simulink model "Channelizer_HLS_testbench"  (R2024a)
settings: Solver=VariableStepAuto  StartTime=0.0  StopTime=512  RelTol=1e-3
undefined symbols (not defined in the file): cyclicshift, permutei, permuteo, S, vsva2197, xcvc1902
libraries: aieUtilities x71, dspsrcs4 x23, hlsBasic x3, vmcUtilities x1
settings Model: Creator=robg  LastModifiedBy=robg
settings DebuggingCC: UnconnectedInputMsg=warning  UnconnectedOutputMsg=warning  UnconnectedLineMsg=warning
settings ModelReferenceCC: EnableRefExpFcnMdlSchedulingChecks=on
settings RTWCC: GPUComputeCapability=3.5  DLArmComputeVersion=19.05

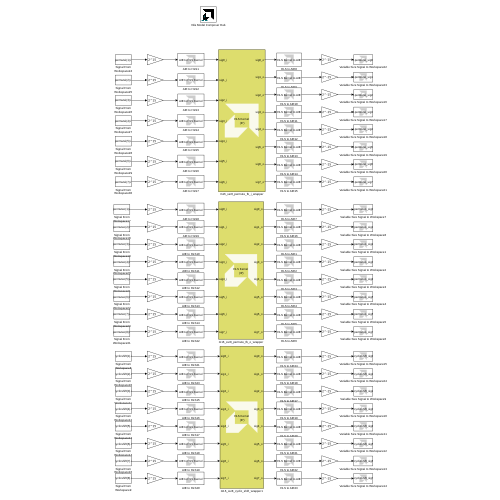
[thumbnail: Simulink's stored preview of the top-level diagram]
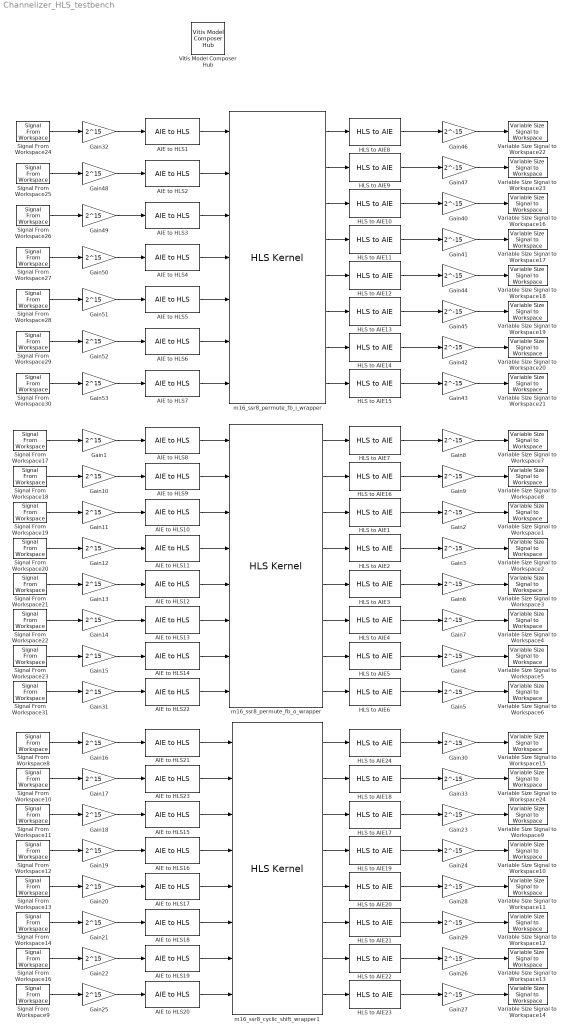
== system Channelizer_HLS_testbench ==
  AIE to HLS{1..23} (23 alike) : aieUtilities/AIE to HLS  OutputType=ufix128  OutputSize=1  AllowMultiRate=off  InputType=int8
  Gain{1,10..22,25,31..32,48..53} (23 alike) : Gain  Gain=2^15  OutDataTypeStr=int16
  Gain{2..9,23..24,26..30,33,40..47} (24 alike) : Gain  Gain=2^-15  OutDataTypeStr=double
  HLS to AIE{1..24} (24 alike) : aieUtilities/HLS to AIE  OutputType=cint16  OutputSize=4  AllowMultiRate=off  InputType=cint16
  Signal From Workspace10 : dspsrcs4/Signal From Workspace  X=cyclicshift(2).i  Ts=1  nsamps=4  OutputAfterFinalValue=Setting to zero  ignoreOrWarnInputAndFrameLengths=off  OutputFrames=off
  Signal From Workspace11 : dspsrcs4/Signal From Workspace  X=cyclicshift(3).i  Ts=1  nsamps=4  OutputAfterFinalValue=Setting to zero  ignoreOrWarnInputAndFrameLengths=off  OutputFrames=off
  Signal From Workspace12 : dspsrcs4/Signal From Workspace  X=cyclicshift(4).i  Ts=1  nsamps=4  OutputAfterFinalValue=Setting to zero  ignoreOrWarnInputAndFrameLengths=off  OutputFrames=off
  Signal From Workspace13 : dspsrcs4/Signal From Workspace  X=cyclicshift(5).i  Ts=1  nsamps=4  OutputAfterFinalValue=Setting to zero  ignoreOrWarnInputAndFrameLengths=off  OutputFrames=off
  Signal From Workspace14 : dspsrcs4/Signal From Workspace  X=cyclicshift(6).i  Ts=1  nsamps=4  OutputAfterFinalValue=Setting to zero  ignoreOrWarnInputAndFrameLengths=off  OutputFrames=off
  Signal From Workspace16 : dspsrcs4/Signal From Workspace  X=cyclicshift(7).i  Ts=1  nsamps=4  OutputAfterFinalValue=Setting to zero  ignoreOrWarnInputAndFrameLengths=off  OutputFrames=off
  Signal From Workspace17 : dspsrcs4/Signal From Workspace  X=permuteo(1).i  Ts=1  nsamps=4  OutputAfterFinalValue=Setting to zero  ignoreOrWarnInputAndFrameLengths=off  OutputFrames=off
  Signal From Workspace18 : dspsrcs4/Signal From Workspace  X=permuteo(2).i  Ts=1  nsamps=4  OutputAfterFinalValue=Setting to zero  ignoreOrWarnInputAndFrameLengths=off  OutputFrames=off
  Signal From Workspace19 : dspsrcs4/Signal From Workspace  X=permuteo(3).i  Ts=1  nsamps=4  OutputAfterFinalValue=Setting to zero  ignoreOrWarnInputAndFrameLengths=off  OutputFrames=off
  Signal From Workspace20 : dspsrcs4/Signal From Workspace  X=permuteo(4).i  Ts=1  nsamps=4  OutputAfterFinalValue=Setting to zero  ignoreOrWarnInputAndFrameLengths=off  OutputFrames=off
  Signal From Workspace21 : dspsrcs4/Signal From Workspace  X=permuteo(5).i  Ts=1  nsamps=4  OutputAfterFinalValue=Setting to zero  ignoreOrWarnInputAndFrameLengths=off  OutputFrames=off
  Signal From Workspace22 : dspsrcs4/Signal From Workspace  X=permuteo(6).i  Ts=1  nsamps=4  OutputAfterFinalValue=Setting to zero  ignoreOrWarnInputAndFrameLengths=off  OutputFrames=off
  Signal From Workspace23 : dspsrcs4/Signal From Workspace  X=permuteo(7).i  Ts=1  nsamps=4  OutputAfterFinalValue=Setting to zero  ignoreOrWarnInputAndFrameLengths=off  OutputFrames=off
  Signal From Workspace24 : dspsrcs4/Signal From Workspace  X=permutei(1).i  Ts=1  nsamps=4  OutputAfterFinalValue=Setting to zero  ignoreOrWarnInputAndFrameLengths=off  OutputFrames=off
  Signal From Workspace25 : dspsrcs4/Signal From Workspace  X=permutei(2).i  Ts=1  nsamps=4  OutputAfterFinalValue=Setting to zero  ignoreOrWarnInputAndFrameLengths=off  OutputFrames=off
  Signal From Workspace26 : dspsrcs4/Signal From Workspace  X=permutei(3).i  Ts=1  nsamps=4  OutputAfterFinalValue=Setting to zero  ignoreOrWarnInputAndFrameLengths=off  OutputFrames=off
  Signal From Workspace27 : dspsrcs4/Signal From Workspace  X=permutei(4).i  Ts=1  nsamps=4  OutputAfterFinalValue=Setting to zero  ignoreOrWarnInputAndFrameLengths=off  OutputFrames=off
  Signal From Workspace28 : dspsrcs4/Signal From Workspace  X=permutei(5).i  Ts=1  nsamps=4  OutputAfterFinalValue=Setting to zero  ignoreOrWarnInputAndFrameLengths=off  OutputFrames=off
  Signal From Workspace29 : dspsrcs4/Signal From Workspace  X=permutei(6).i  Ts=1  nsamps=4  OutputAfterFinalValue=Setting to zero  ignoreOrWarnInputAndFrameLengths=off  OutputFrames=off
  Signal From Workspace30 : dspsrcs4/Signal From Workspace  X=permutei(7).i  Ts=1  nsamps=4  OutputAfterFinalValue=Setting to zero  ignoreOrWarnInputAndFrameLengths=off  OutputFrames=off
  Signal From Workspace31 : dspsrcs4/Signal From Workspace  X=permuteo(8).i  Ts=1  nsamps=4  OutputAfterFinalValue=Setting to zero  ignoreOrWarnInputAndFrameLengths=off  OutputFrames=off
  Signal From Workspace8 : dspsrcs4/Signal From Workspace  X=cyclicshift(1).i  Ts=1  nsamps=4  OutputAfterFinalValue=Setting to zero  ignoreOrWarnInputAndFrameLengths=off  OutputFrames=off
  Signal From Workspace9 : dspsrcs4/Signal From Workspace  X=cyclicshift(8).i  Ts=1  nsamps=4  OutputAfterFinalValue=Setting to zero  ignoreOrWarnInputAndFrameLengths=off  OutputFrames=off
  Variable Size Signal to Workspace1 : aieUtilities/Variable Size Signal to Workspace  VariableNameMask=permuteo_sig2_o
  Variable Size Signal to Workspace10 : aieUtilities/Variable Size Signal to Workspace  VariableNameMask=cyclicshift_sig3_o
  Variable Size Signal to Workspace11 : aieUtilities/Variable Size Signal to Workspace  VariableNameMask=cyclicshift_sig4_o
  Variable Size Signal to Workspace12 : aieUtilities/Variable Size Signal to Workspace  VariableNameMask=cyclicshift_sig5_o
  Variable Size Signal to Workspace13 : aieUtilities/Variable Size Signal to Workspace  VariableNameMask=cyclicshift_sig6_o
  Variable Size Signal to Workspace14 : aieUtilities/Variable Size Signal to Workspace  VariableNameMask=cyclicshift_sig7_o
  Variable Size Signal to Workspace15 : aieUtilities/Variable Size Signal to Workspace  VariableNameMask=cyclicshift_sig0_o
  Variable Size Signal to Workspace16 : aieUtilities/Variable Size Signal to Workspace  VariableNameMask=permutei_sig2_o
  Variable Size Signal to Workspace17 : aieUtilities/Variable Size Signal to Workspace  VariableNameMask=permutei_sig3_o
  Variable Size Signal to Workspace18 : aieUtilities/Variable Size Signal to Workspace  VariableNameMask=permutei_sig4_o
  Variable Size Signal to Workspace19 : aieUtilities/Variable Size Signal to Workspace  VariableNameMask=permutei_sig5_o
  Variable Size Signal to Workspace2 : aieUtilities/Variable Size Signal to Workspace  VariableNameMask=permuteo_sig3_o
  Variable Size Signal to Workspace20 : aieUtilities/Variable Size Signal to Workspace  VariableNameMask=permutei_sig6_o
  Variable Size Signal to Workspace21 : aieUtilities/Variable Size Signal to Workspace  VariableNameMask=permutei_sig7_o
  Variable Size Signal to Workspace22 : aieUtilities/Variable Size Signal to Workspace  VariableNameMask=permutei_sig0_o
  Variable Size Signal to Workspace23 : aieUtilities/Variable Size Signal to Workspace  VariableNameMask=permutei_sig1_o
  Variable Size Signal to Workspace24 : aieUtilities/Variable Size Signal to Workspace  VariableNameMask=cyclicshift_sig1_o
  Variable Size Signal to Workspace3 : aieUtilities/Variable Size Signal to Workspace  VariableNameMask=permuteo_sig4_o
  Variable Size Signal to Workspace4 : aieUtilities/Variable Size Signal to Workspace  VariableNameMask=permuteo_sig5_o
  Variable Size Signal to Workspace5 : aieUtilities/Variable Size Signal to Workspace  VariableNameMask=permuteo_sig6_o
  Variable Size Signal to Workspace6 : aieUtilities/Variable Size Signal to Workspace  VariableNameMask=permuteo_sig7_o
  Variable Size Signal to Workspace7 : aieUtilities/Variable Size Signal to Workspace  VariableNameMask=permuteo_sig0_o
  Variable Size Signal to Workspace8 : aieUtilities/Variable Size Signal to Workspace  VariableNameMask=permuteo_sig1_o
  Variable Size Signal to Workspace9 : aieUtilities/Variable Size Signal to Workspace  VariableNameMask=cyclicshift_sig2_o
  Vitis Model Composer Hub : vmcUtilities/Vitis Model Composer Hub  Tag=genX  CodeGeneration=off  StartColumn=1  NumberOfColumns=1  TargetDirectory=./code  exportDesign=off  analyzeDesign=off  validateDesignOnHw=off  ExportType=AI Engines  IpVendor=xilinx.com  IpLibrary=hls  IpVersion=1.0  IpHWLanguage=Verilog  AieCompilerOptions={}  AieSimulatorOptions={}  CreateTestbench=off  TestbenchStackSize=10  RunRtlSim=off  RunCSim=off  RunAieSim=off  AieSimTimeout=50000  RunAieSimProfiling=off  LaunchVitisAnalyzer=off  PlotOutput=off  RunX86Sim=off  X86SimTimeout=10  GenHwImage=off  GenLibadfXo=off  GenHwValidationCode=off  PlatformType=Not Specified  HwSystemType=Baremetal  HwValidationTarget=hw  ProjDevice=xcvc1902-vsva2197-1LP-e-S  ProjDevicePart=xcvc1902-vsva2197-1LP-e-S  AIEType=AIE  SamplePeriod=-1  ClockFrequency=200  DataPathParallelism=1  xilinxfamily=versalaicore  part=xcvc1902  speed=-1LP-e-S  package=vsva2197  directory=./netlist  testbench=off  incr_netlist=off  synthesis_tool=Vivado  clock_wrapper=Clock Enables  dbl_ovrd=According to Block Masks  dcm_input_clock_period=10  sysclk_period=10  simulink_period=1  eval_field=0  LogFileName=''  NThreads=4
  m16_ssr8_cyclic_shift_wrapper1 : hlsBasic/HLS Kernel  PortNames={'return'; 'sig0_i'; 'sig1_i'; 'sig2_i'; 'sig3_i'; 'sig4_i'; 'sig5_i'; 'sig6_i'; 'sig7_i'; 'sig0_o'; 'sig1_o'; 'sig2_o'; 'sig3_o'; 'sig4_o'; 'sig5_o'; 'sig6_o'; 'sig7_o'}  PortSerializedTypes={'{Bv}'; '{R{Thls::stream{2{t{Tap_uint{1{t{}128}}}}{t{}0}}}}'; '{R{Thls::stream{2{t{Tap_uint{1{t{}128}}}}{t{}0}}}}'; '{R{Thls::stream{2{t{Tap_uint{1{t{}128}}}}{t{}0}}}}'; '{R{Thls::stream{2{t{Tap_uint{1{t{}128}}}}{t{}0}}}}'; '{R{Thls::stream{2{t{Tap_uint{1{t{}128}}}}{t{}0}}}}'; '{R{Thls::stream{2{t{Tap_uint{1{t{}128}}}}{t{}0}}}}'; '{R{Thls::stream{2{t{Tap_uint{1{t{}128}}}}{t{}0}}}}'; '{R{Thls::stream{2{t{Tap_uint{1{t{}128}}}}{t{}0}}}}'; '{R{Thls::stream{2{t{Tap_uint{1{t{}128}}}}{t{}0}}}}'; '{R{Thls::stream{2{t{Tap_uint{1{t{}128}}}}{t{}0}}}}'; '{R{Thls::stream{2{t{Tap_uint{1{t{}128}}}}{t{}0}}}}'; '{R{Thls::stream{2{t{Tap_uint{1{t{}128}}}}{t{}0}}}}'; '{R{Thls::stream{2{t{Tap_uint{1{t{}128}}}}{t{}0}}}}'; '{R{Thls::stream{2{t{Tap_uint{1{t{}128}}}}{t{}0}}}}'; '{R{Thls::stream{2{t{Tap_uint{1{t{}128}}}}{t{}0}}}}'; '{R{Thls::stream{2{t{Tap_uint{1{t{}128}}}}{t{}0}}}}'}  FunctionTemplateSpecKind=none  FunctionTemplateParamNames={}  FunctionTemplateParamKinds={}  FunctionTemplateParamTypes={}  FunctionTemplateParamValues={}  PortSynchronicities={'auto'; 'auto'; 'auto'; 'auto'; 'auto'; 'auto'; 'auto'; 'auto'; 'auto'; 'auto'; 'auto'; 'auto'; 'auto'; 'auto'; 'auto'; 'auto'}  PortSignalSizes={0.000000000000000000e+00; 0.000000000000000000e+00; 0.000000000000000000e+00; 0.000000000000000000e+00; 0.000000000000000000e+00; 0.000000000000000000e+00; 0.000000000000000000e+00; 0.000000000000000000e+00; 1.000000000000000000e+00; 1.000000000000000000e+00; 1.000000000000000000e+00; 1.000000000000000000e+00; 1.000000000000000000e+00; 1.000000000000000000e+00; 1.000000000000000000e+00; 1.000000000000000000e+00}  PortParameterValues={}  PortAttributesTable={ 'Input', 'sig0_i', 'hls::stream< ap_uint< 128 >, 0 > &', '', ''; 'Input', 'sig1_i', 'hls::stream< ap_uint< 128 >, 0 > &', '', ''; 'Input', 'sig2_i', 'hls::stream< ap_uint< 128 >, 0 > &', '', ''; 'Input', 'sig3_i', 'hls::stream< ap_uint< 128 >, 0 > &', '', ''; 'Input', 'sig4_i', 'hls::stream< ap_uint< 128 >, 0 > &', '', ''; 'Input', 'sig5_i', 'hls::stream< ap_uint< 128 >, 0 > &', '', ''; 'Input', 'sig6_i', 'hls::stream< ap_uint< 128 >, 0 > &', '', ''; 'Input', 'sig7_i', 'hls::stream< ap_uint< 128 >, 0 > &', '', ''; 'Output', 'sig0_o', 'hls::stream< ap_uint< 128 >, 0 > &', '', '1'; 'Output', 'sig1_o', 'hls::stream< ap_uint< 128 >, 0 > &', '', '1'; 'Output', 'sig2_o', 'hls::stream< ap_uint< 128 >, 0 > &', '', '1'; 'Output', 'sig3_o', 'hls::stream< ap_uint< 128 >, 0 > &', '', '1'; 'Output', 'sig4_o', 'hls::stream< ap_uint< 128 >, 0 > &', '', '1'; 'Output', 'sig5_o', 'hls::stream< ap_uint< 128 >, 0 > &', '', '1'; 'Output', 'sig6_o', 'hls::stream< ap_uint< 128 >, 0 > &', '', '1'; 'Output', 'sig7_o', 'hls::stream< ap_uint< 128 >, 0 > &', '', '1' }  PortAttributesEnablement={'off', 'off', 'off', 'off', 'off';'off', 'off', 'off', 'off', 'off';'off', 'off', 'off', 'off', 'off';'off', 'off', 'off', 'off', 'off';'off', 'off', 'off', 'off', 'off';'off', 'off', 'off', 'off', 'off';'off', 'off', 'off', 'off', 'off';'off', 'off', 'off', 'off', 'off';'off', 'off', 'off', 'off', 'on';'off', 'off', 'off', 'off', 'on';'off', 'off', 'off', 'off', 'on';'off', 'off', 'off', 'off', 'on';'off', 'off', 'off', 'off', 'on';'off', 'off', 'off', 'off', 'on';'off', 'off', 'off', 'off', 'on';'off', 'off', 'off', 'off', 'on'}  PortParametersTable={}  SampleTime=-1  PortDirectionTable={ 'sig0_i', 'hls::stream< ap_uint< 128 >, 0 > &', 'Input', 'Port'; 'sig1_i', 'hls::stream< ap_uint< 128 >, 0 > &', 'Input', 'Port'; 'sig2_i', 'hls::stream< ap_uint< 128 >, 0 > &', 'Input', 'Port'; 'sig3_i', 'hls::stream< ap_uint< 128 >, 0 > &', 'Input', 'Port'; 'sig4_i', 'hls::stream< ap_uint< 128 >, 0 > &', 'Input', 'Port'; 'sig5_i', 'hls::stream< ap_uint< 128 >, 0 > &', 'Input', 'Port'; 'sig6_i', 'hls::stream< ap_uint< 128 >, 0 > &', 'Input', 'Port'; 'sig7_i', 'hls::stream< ap_uint< 128 >, 0 > &', 'Input', 'Port'; 'sig0_o', 'hls::stream< ap_uint< 128 >, 0 > &', 'Output', 'Port'; 'sig1_o', 'hls::stream< ap_uint< 128 >, 0 > &', 'Output', 'Port'; 'sig2_o', 'hls::stream< ap_uint< 128 >, 0 > &', 'Output', 'Port'; 'sig3_o', 'hls::stream< ap_uint< 128 >, 0 > &', 'Output', 'Port'; 'sig4_o', 'hls::stream< ap_uint< 128 >, 0 > &', 'Output', 'Port'; 'sig5_o', 'hls::stream< ap_uint< 128 >, 0 > &', 'Output', 'Port'; 'sig6_o', 'hls::stream< ap_uint< 128 >, 0 > &', 'Output', 'Port'; 'sig7_o', 'hls::stream< ap_uint< 128 >, 0 > &', 'Output', 'Port' }  FunctionTemplateParams={}  FunctionTemplateParamsEnables={}  FunctionTemplateParamsVisible=off  FunctionDeclTypeOptions=C[1 1]@t7@<empty>  PortDirectionTabVisible=on  ArgDirections={1.000000000000000000e+00; 1.000000000000000000e+00; 1.000000000000000000e+00; 1.000000000000000000e+00; 1.000000000000000000e+00; 1.000000000000000000e+00; 1.000000000000000000e+00; 1.000000000000000000e+00; 2.000000000000000000e+00; 2.000000000000000000e+00; 2.000000000000000000e+00; 2.000000000000000000e+00; 2.000000000000000000e+00; 2.000000000000000000e+00; 2.000000000000000000e+00; 2.000000000000000000e+00}  ArgInterfaceTypes={1.000000000000000000e+00; 1.000000000000000000e+00; 1.000000000000000000e+00; 1.000000000000000000e+00; 1.000000000000000000e+00; 1.000000000000000000e+00; 1.000000000000000000e+00; 1.000000000000000000e+00; 1.000000000000000000e+00; 1.000000000000000000e+00; 1.000000000000000000e+00; 1.000000000000000000e+00; 1.000000000000000000e+00; 1.000000000000000000e+00; 1.000000000000000000e+00; 1.000000000000000000e+00}  FunctionIndex=1  FormalArgDecls={'hls::stream< ap_uint< 128 >, 0 > & sig0_i', 'hls::stream< ap_uint< 128 >, 0 > & sig1_i', 'hls::stream< ap_uint< 128 >, 0 > & sig2_i', 'hls::stream< ap_uint< 128 >, 0 > & sig3_i', 'hls::stream< ap_uint< 128 >, 0 > & sig4_i', 'hls::stream< ap_uint< 128 >, 0 > & sig5_i', 'hls::stream< ap_uint< 128 >, 0 > & sig6_i', 'hls::stream< ap_uint< 128 >, 0 > & sig7_i', 'hls::stream< ap_uint< 128 >, 0 > & sig0_o', 'hls::stream< ap_uint< 128 >, 0 > & sig1_o', 'hls::stream< ap_uint< 128 >, 0 > & sig2_o', 'hls::stream< ap_uint< 128 >, 0 > & sig3_o', 'hls::stream< ap_uint< 128 >, 0 > & sig4_o', 'hls::stream< ap_uint< 128 >, 0 > & sig5_o', 'hls::stream< ap_uint< 128 >, 0 > & sig6_o', 'hls::stream< ap_uint< 128 >, 0 > & sig7_o'}  SimLibPath=''  FunctionTabVisible=on  FunctionDescription=void m16_ssr8_cyclic_shift_wrapper(hls::stream< ap_uint< 128 >, 0 > & sig0_i, hls::stream< ap_uint< 128 >, 0 > & sig1_i, hls::stream< ap_uint< 128 >, 0 > & sig2_i, hls::stream< ap_uint< 128 >, 0 > & sig3_i, hls::stream< ap_uint< 128 >, 0 > & sig4_i, hls::stream< ap_uint< 128 >, 0 > & sig5_i, hls::stream< ap_uint< 128 >, 0 > & sig6_i, hls::stream< ap_uint< 128 >, 0 > & sig7_i, hls::stream< ap_uint< 128 >, 0 > & sig0_o, hls::stream< ap_uint< 128 >, 0 > & sig1_o, hls::stream< ap_uint< 128 >, 0 > & sig2_o, hls::stream< ap_uint< 128 >, 0 > & sig3_o, hls::stream< ap_uint< 128 >, 0 > & sig4_o, hls::stream< ap_uint< 128 >, 0 > & sig5_o, hls::stream< ap_uint< 128 >, 0 > & sig6_o, hls::stream< ap_uint< 128 >, 0 > & sig7_o)  blockJsonConstraints=[]  deprecateConstraints=0  KernelHeaderFile=/proj/xcoswmktg/robg/git/designs/channelizer/hls/m16_ssr8_cyclic_shift/m16_ssr8_cyclic_shift.h  KernelFunction=m16_ssr8_cyclic_shift_wrapper  KernelFunctionSelect=<empty>  KernelSourceFile=/proj/xcoswmktg/robg/git/designs/channelizer/hls/m16_ssr8_cyclic_shift/m16_ssr8_cyclic_shift.cpp  KernelSearchPaths={}  PreProcOptions={}
  m16_ssr8_permute_fb_i_wrapper : hlsBasic/HLS Kernel  PortNames={'return'; 'sig0_i'; 'sig1_i'; 'sig2_i'; 'sig3_i'; 'sig4_i'; 'sig5_i'; 'sig6_i'; 'sig0_o'; 'sig1_o'; 'sig2_o'; 'sig3_o'; 'sig4_o'; 'sig5_o'; 'sig6_o'; 'sig7_o'}  PortSerializedTypes={'{Bv}'; '{R{Thls::stream{2{t{Tap_uint{1{t{}128}}}}{t{}0}}}}'; '{R{Thls::stream{2{t{Tap_uint{1{t{}128}}}}{t{}0}}}}'; '{R{Thls::stream{2{t{Tap_uint{1{t{}128}}}}{t{}0}}}}'; '{R{Thls::stream{2{t{Tap_uint{1{t{}128}}}}{t{}0}}}}'; '{R{Thls::stream{2{t{Tap_uint{1{t{}128}}}}{t{}0}}}}'; '{R{Thls::stream{2{t{Tap_uint{1{t{}128}}}}{t{}0}}}}'; '{R{Thls::stream{2{t{Tap_uint{1{t{}128}}}}{t{}0}}}}'; '{R{Thls::stream{2{t{Tap_uint{1{t{}128}}}}{t{}0}}}}'; '{R{Thls::stream{2{t{Tap_uint{1{t{}128}}}}{t{}0}}}}'; '{R{Thls::stream{2{t{Tap_uint{1{t{}128}}}}{t{}0}}}}'; '{R{Thls::stream{2{t{Tap_uint{1{t{}128}}}}{t{}0}}}}'; '{R{Thls::stream{2{t{Tap_uint{1{t{}128}}}}{t{}0}}}}'; '{R{Thls::stream{2{t{Tap_uint{1{t{}128}}}}{t{}0}}}}'; '{R{Thls::stream{2{t{Tap_uint{1{t{}128}}}}{t{}0}}}}'; '{R{Thls::stream{2{t{Tap_uint{1{t{}128}}}}{t{}0}}}}'}  FunctionTemplateSpecKind=none  FunctionTemplateParamNames={}  FunctionTemplateParamKinds={}  FunctionTemplateParamTypes={}  FunctionTemplateParamValues={}  PortSynchronicities={'auto'; 'auto'; 'auto'; 'auto'; 'auto'; 'auto'; 'auto'; 'auto'; 'auto'; 'auto'; 'auto'; 'auto'; 'auto'; 'auto'; 'auto'}  PortSignalSizes={0.000000000000000000e+00; 0.000000000000000000e+00; 0.000000000000000000e+00; 0.000000000000000000e+00; 0.000000000000000000e+00; 0.000000000000000000e+00; 0.000000000000000000e+00; 1.000000000000000000e+00; 1.000000000000000000e+00; 1.000000000000000000e+00; 1.000000000000000000e+00; 1.000000000000000000e+00; 1.000000000000000000e+00; 1.000000000000000000e+00; 1.000000000000000000e+00}  PortParameterValues={}  PortAttributesTable={ 'Input', 'sig0_i', 'hls::stream< ap_uint< 128 >, 0 > &', '', ''; 'Input', 'sig1_i', 'hls::stream< ap_uint< 128 >, 0 > &', '', ''; 'Input', 'sig2_i', 'hls::stream< ap_uint< 128 >, 0 > &', '', ''; 'Input', 'sig3_i', 'hls::stream< ap_uint< 128 >, 0 > &', '', ''; 'Input', 'sig4_i', 'hls::stream< ap_uint< 128 >, 0 > &', '', ''; 'Input', 'sig5_i', 'hls::stream< ap_uint< 128 >, 0 > &', '', ''; 'Input', 'sig6_i', 'hls::stream< ap_uint< 128 >, 0 > &', '', ''; 'Output', 'sig0_o', 'hls::stream< ap_uint< 128 >, 0 > &', '', '1'; 'Output', 'sig1_o', 'hls::stream< ap_uint< 128 >, 0 > &', '', '1'; 'Output', 'sig2_o', 'hls::stream< ap_uint< 128 >, 0 > &', '', '1'; 'Output', 'sig3_o', 'hls::stream< ap_uint< 128 >, 0 > &', '', '1'; 'Output', 'sig4_o', 'hls::stream< ap_uint< 128 >, 0 > &', '', '1'; 'Output', 'sig5_o', 'hls::stream< ap_uint< 128 >, 0 > &', '', '1'; 'Output', 'sig6_o', 'hls::stream< ap_uint< 128 >, 0 > &', '', '1'; 'Output', 'sig7_o', 'hls::stream< ap_uint< 128 >, 0 > &', '', '1' }  PortAttributesEnablement={'off', 'off', 'off', 'off', 'off';'off', 'off', 'off', 'off', 'off';'off', 'off', 'off', 'off', 'off';'off', 'off', 'off', 'off', 'off';'off', 'off', 'off', 'off', 'off';'off', 'off', 'off', 'off', 'off';'off', 'off', 'off', 'off', 'off';'off', 'off', 'off', 'off', 'on';'off', 'off', 'off', 'off', 'on';'off', 'off', 'off', 'off', 'on';'off', 'off', 'off', 'off', 'on';'off', 'off', 'off', 'off', 'on';'off', 'off', 'off', 'off', 'on';'off', 'off', 'off', 'off', 'on';'off', 'off', 'off', 'off', 'on'}  PortParametersTable={}  SampleTime=-1  PortDirectionTable={ 'sig0_i', 'hls::stream< ap_uint< 128 >, 0 > &', 'Input', 'Port'; 'sig1_i', 'hls::stream< ap_uint< 128 >, 0 > &', 'Input', 'Port'; 'sig2_i', 'hls::stream< ap_uint< 128 >, 0 > &', 'Input', 'Port'; 'sig3_i', 'hls::stream< ap_uint< 128 >, 0 > &', 'Input', 'Port'; 'sig4_i', 'hls::stream< ap_uint< 128 >, 0 > &', 'Input', 'Port'; 'sig5_i', 'hls::stream< ap_uint< 128 >, 0 > &', 'Input', 'Port'; 'sig6_i', 'hls::stream< ap_uint< 128 >, 0 > &', 'Input', 'Port'; 'sig0_o', 'hls::stream< ap_uint< 128 >, 0 > &', 'Output', 'Port'; 'sig1_o', 'hls::stream< ap_uint< 128 >, 0 > &', 'Output', 'Port'; 'sig2_o', 'hls::stream< ap_uint< 128 >, 0 > &', 'Output', 'Port'; 'sig3_o', 'hls::stream< ap_uint< 128 >, 0 > &', 'Output', 'Port'; 'sig4_o', 'hls::stream< ap_uint< 128 >, 0 > &', 'Output', 'Port'; 'sig5_o', 'hls::stream< ap_uint< 128 >, 0 > &', 'Output', 'Port'; 'sig6_o', 'hls::stream< ap_uint< 128 >, 0 > &', 'Output', 'Port'; 'sig7_o', 'hls::stream< ap_uint< 128 >, 0 > &', 'Output', 'Port' }  FunctionTemplateParams={}  FunctionTemplateParamsEnables={}  FunctionTemplateParamsVisible=off  FunctionDeclTypeOptions=C[1 1]@t7@<empty>  PortDirectionTabVisible=on  ArgDirections={1.000000000000000000e+00; 1.000000000000000000e+00; 1.000000000000000000e+00; 1.000000000000000000e+00; 1.000000000000000000e+00; 1.000000000000000000e+00; 1.000000000000000000e+00; 2.000000000000000000e+00; 2.000000000000000000e+00; 2.000000000000000000e+00; 2.000000000000000000e+00; 2.000000000000000000e+00; 2.000000000000000000e+00; 2.000000000000000000e+00; 2.000000000000000000e+00}  ArgInterfaceTypes={1.000000000000000000e+00; 1.000000000000000000e+00; 1.000000000000000000e+00; 1.000000000000000000e+00; 1.000000000000000000e+00; 1.000000000000000000e+00; 1.000000000000000000e+00; 1.000000000000000000e+00; 1.000000000000000000e+00; 1.000000000000000000e+00; 1.000000000000000000e+00; 1.000000000000000000e+00; 1.000000000000000000e+00; 1.000000000000000000e+00; 1.000000000000000000e+00}  FunctionIndex=1  FormalArgDecls={'hls::stream< ap_uint< 128 >, 0 > & sig0_i', 'hls::stream< ap_uint< 128 >, 0 > & sig1_i', 'hls::stream< ap_uint< 128 >, 0 > & sig2_i', 'hls::stream< ap_uint< 128 >, 0 > & sig3_i', 'hls::stream< ap_uint< 128 >, 0 > & sig4_i', 'hls::stream< ap_uint< 128 >, 0 > & sig5_i', 'hls::stream< ap_uint< 128 >, 0 > & sig6_i', 'hls::stream< ap_uint< 128 >, 0 > & sig0_o', 'hls::stream< ap_uint< 128 >, 0 > & sig1_o', 'hls::stream< ap_uint< 128 >, 0 > & sig2_o', 'hls::stream< ap_uint< 128 >, 0 > & sig3_o', 'hls::stream< ap_uint< 128 >, 0 > & sig4_o', 'hls::stream< ap_uint< 128 >, 0 > & sig5_o', 'hls::stream< ap_uint< 128 >, 0 > & sig6_o', 'hls::stream< ap_uint< 128 >, 0 > & sig7_o'}  SimLibPath=''  FunctionTabVisible=on  FunctionDescription=void m16_ssr8_permute_fb_i_wrapper(hls::stream< ap_uint< 128 >, 0 > & sig0_i, hls::stream< ap_uint< 128 >, 0 > & sig1_i, hls::stream< ap_uint< 128 >, 0 > & sig2_i, hls::stream< ap_uint< 128 >, 0 > & sig3_i, hls::stream< ap_uint< 128 >, 0 > & sig4_i, hls::stream< ap_uint< 128 >, 0 > & sig5_i, hls::stream< ap_uint< 128 >, 0 > & sig6_i, hls::stream< ap_uint< 128 >, 0 > & sig0_o, hls::stream< ap_uint< 128 >, 0 > & sig1_o, hls::stream< ap_uint< 128 >, 0 > & sig2_o, hls::stream< ap_uint< 128 >, 0 > & sig3_o, hls::stream< ap_uint< 128 >, 0 > & sig4_o, hls::stream< ap_uint< 128 >, 0 > & sig5_o, hls::stream< ap_uint< 128 >, 0 > & sig6_o, hls::stream< ap_uint< 128 >, 0 > & sig7_o)  blockJsonConstraints=[]  deprecateConstraints=0  KernelHeaderFile=/proj/xcoswmktg/robg/git/designs/channelizer/hls/m16_ssr8_permute_fb_i/m16_ssr8_permute_fb_i.h  KernelFunction=m16_ssr8_permute_fb_i_wrapper  KernelFunctionSelect=<empty>  KernelSourceFile=/proj/xcoswmktg/robg/git/designs/channelizer/hls/m16_ssr8_permute_fb_i/m16_ssr8_permute_fb_i.cpp  KernelSearchPaths={}  PreProcOptions={}
  m16_ssr8_permute_fb_o_wrapper : hlsBasic/HLS Kernel  PortNames={'return'; 'sig0_i'; 'sig1_i'; 'sig2_i'; 'sig3_i'; 'sig4_i'; 'sig5_i'; 'sig6_i'; 'sig7_i'; 'sig0_o'; 'sig1_o'; 'sig2_o'; 'sig3_o'; 'sig4_o'; 'sig5_o'; 'sig6_o'; 'sig7_o'}  PortSerializedTypes={'{Bv}'; '{R{Thls::stream{2{t{Tap_uint{1{t{}128}}}}{t{}0}}}}'; '{R{Thls::stream{2{t{Tap_uint{1{t{}128}}}}{t{}0}}}}'; '{R{Thls::stream{2{t{Tap_uint{1{t{}128}}}}{t{}0}}}}'; '{R{Thls::stream{2{t{Tap_uint{1{t{}128}}}}{t{}0}}}}'; '{R{Thls::stream{2{t{Tap_uint{1{t{}128}}}}{t{}0}}}}'; '{R{Thls::stream{2{t{Tap_uint{1{t{}128}}}}{t{}0}}}}'; '{R{Thls::stream{2{t{Tap_uint{1{t{}128}}}}{t{}0}}}}'; '{R{Thls::stream{2{t{Tap_uint{1{t{}128}}}}{t{}0}}}}'; '{R{Thls::stream{2{t{Tap_uint{1{t{}128}}}}{t{}0}}}}'; '{R{Thls::stream{2{t{Tap_uint{1{t{}128}}}}{t{}0}}}}'; '{R{Thls::stream{2{t{Tap_uint{1{t{}128}}}}{t{}0}}}}'; '{R{Thls::stream{2{t{Tap_uint{1{t{}128}}}}{t{}0}}}}'; '{R{Thls::stream{2{t{Tap_uint{1{t{}128}}}}{t{}0}}}}'; '{R{Thls::stream{2{t{Tap_uint{1{t{}128}}}}{t{}0}}}}'; '{R{Thls::stream{2{t{Tap_uint{1{t{}128}}}}{t{}0}}}}'; '{R{Thls::stream{2{t{Tap_uint{1{t{}128}}}}{t{}0}}}}'}  FunctionTemplateSpecKind=none  FunctionTemplateParamNames={}  FunctionTemplateParamKinds={}  FunctionTemplateParamTypes={}  FunctionTemplateParamValues={}  PortSynchronicities={'auto'; 'auto'; 'auto'; 'auto'; 'auto'; 'auto'; 'auto'; 'auto'; 'auto'; 'auto'; 'auto'; 'auto'; 'auto'; 'auto'; 'auto'; 'auto'}  PortSignalSizes={0.000000000000000000e+00; 0.000000000000000000e+00; 0.000000000000000000e+00; 0.000000000000000000e+00; 0.000000000000000000e+00; 0.000000000000000000e+00; 0.000000000000000000e+00; 0.000000000000000000e+00; 1.000000000000000000e+00; 1.000000000000000000e+00; 1.000000000000000000e+00; 1.000000000000000000e+00; 1.000000000000000000e+00; 1.000000000000000000e+00; 1.000000000000000000e+00; 1.000000000000000000e+00}  PortParameterValues={}  PortAttributesTable={ 'Input', 'sig0_i', 'hls::stream< ap_uint< 128 >, 0 > &', '', ''; 'Input', 'sig1_i', 'hls::stream< ap_uint< 128 >, 0 > &', '', ''; 'Input', 'sig2_i', 'hls::stream< ap_uint< 128 >, 0 > &', '', ''; 'Input', 'sig3_i', 'hls::stream< ap_uint< 128 >, 0 > &', '', ''; 'Input', 'sig4_i', 'hls::stream< ap_uint< 128 >, 0 > &', '', ''; 'Input', 'sig5_i', 'hls::stream< ap_uint< 128 >, 0 > &', '', ''; 'Input', 'sig6_i', 'hls::stream< ap_uint< 128 >, 0 > &', '', ''; 'Input', 'sig7_i', 'hls::stream< ap_uint< 128 >, 0 > &', '', ''; 'Output', 'sig0_o', 'hls::stream< ap_uint< 128 >, 0 > &', '', '1'; 'Output', 'sig1_o', 'hls::stream< ap_uint< 128 >, 0 > &', '', '1'; 'Output', 'sig2_o', 'hls::stream< ap_uint< 128 >, 0 > &', '', '1'; 'Output', 'sig3_o', 'hls::stream< ap_uint< 128 >, 0 > &', '', '1'; 'Output', 'sig4_o', 'hls::stream< ap_uint< 128 >, 0 > &', '', '1'; 'Output', 'sig5_o', 'hls::stream< ap_uint< 128 >, 0 > &', '', '1'; 'Output', 'sig6_o', 'hls::stream< ap_uint< 128 >, 0 > &', '', '1'; 'Output', 'sig7_o', 'hls::stream< ap_uint< 128 >, 0 > &', '', '1' }  PortAttributesEnablement={'off', 'off', 'off', 'off', 'off';'off', 'off', 'off', 'off', 'off';'off', 'off', 'off', 'off', 'off';'off', 'off', 'off', 'off', 'off';'off', 'off', 'off', 'off', 'off';'off', 'off', 'off', 'off', 'off';'off', 'off', 'off', 'off', 'off';'off', 'off', 'off', 'off', 'off';'off', 'off', 'off', 'off', 'on';'off', 'off', 'off', 'off', 'on';'off', 'off', 'off', 'off', 'on';'off', 'off', 'off', 'off', 'on';'off', 'off', 'off', 'off', 'on';'off', 'off', 'off', 'off', 'on';'off', 'off', 'off', 'off', 'on';'off', 'off', 'off', 'off', 'on'}  PortParametersTable={}  SampleTime=-1  PortDirectionTable={ 'sig0_i', 'hls::stream< ap_uint< 128 >, 0 > &', 'Input', 'Port'; 'sig1_i', 'hls::stream< ap_uint< 128 >, 0 > &', 'Input', 'Port'; 'sig2_i', 'hls::stream< ap_uint< 128 >, 0 > &', 'Input', 'Port'; 'sig3_i', 'hls::stream< ap_uint< 128 >, 0 > &', 'Input', 'Port'; 'sig4_i', 'hls::stream< ap_uint< 128 >, 0 > &', 'Input', 'Port'; 'sig5_i', 'hls::stream< ap_uint< 128 >, 0 > &', 'Input', 'Port'; 'sig6_i', 'hls::stream< ap_uint< 128 >, 0 > &', 'Input', 'Port'; 'sig7_i', 'hls::stream< ap_uint< 128 >, 0 > &', 'Input', 'Port'; 'sig0_o', 'hls::stream< ap_uint< 128 >, 0 > &', 'Output', 'Port'; 'sig1_o', 'hls::stream< ap_uint< 128 >, 0 > &', 'Output', 'Port'; 'sig2_o', 'hls::stream< ap_uint< 128 >, 0 > &', 'Output', 'Port'; 'sig3_o', 'hls::stream< ap_uint< 128 >, 0 > &', 'Output', 'Port'; 'sig4_o', 'hls::stream< ap_uint< 128 >, 0 > &', 'Output', 'Port'; 'sig5_o', 'hls::stream< ap_uint< 128 >, 0 > &', 'Output', 'Port'; 'sig6_o', 'hls::stream< ap_uint< 128 >, 0 > &', 'Output', 'Port'; 'sig7_o', 'hls::stream< ap_uint< 128 >, 0 > &', 'Output', 'Port' }  FunctionTemplateParams={}  FunctionTemplateParamsEnables={}  FunctionTemplateParamsVisible=off  FunctionDeclTypeOptions=C[1 1]@t7@<empty>  PortDirectionTabVisible=on  ArgDirections={1.000000000000000000e+00; 1.000000000000000000e+00; 1.000000000000000000e+00; 1.000000000000000000e+00; 1.000000000000000000e+00; 1.000000000000000000e+00; 1.000000000000000000e+00; 1.000000000000000000e+00; 2.000000000000000000e+00; 2.000000000000000000e+00; 2.000000000000000000e+00; 2.000000000000000000e+00; 2.000000000000000000e+00; 2.000000000000000000e+00; 2.000000000000000000e+00; 2.000000000000000000e+00}  ArgInterfaceTypes={1.000000000000000000e+00; 1.000000000000000000e+00; 1.000000000000000000e+00; 1.000000000000000000e+00; 1.000000000000000000e+00; 1.000000000000000000e+00; 1.000000000000000000e+00; 1.000000000000000000e+00; 1.000000000000000000e+00; 1.000000000000000000e+00; 1.000000000000000000e+00; 1.000000000000000000e+00; 1.000000000000000000e+00; 1.000000000000000000e+00; 1.000000000000000000e+00; 1.000000000000000000e+00}  FunctionIndex=1  FormalArgDecls={'hls::stream< ap_uint< 128 >, 0 > & sig0_i', 'hls::stream< ap_uint< 128 >, 0 > & sig1_i', 'hls::stream< ap_uint< 128 >, 0 > & sig2_i', 'hls::stream< ap_uint< 128 >, 0 > & sig3_i', 'hls::stream< ap_uint< 128 >, 0 > & sig4_i', 'hls::stream< ap_uint< 128 >, 0 > & sig5_i', 'hls::stream< ap_uint< 128 >, 0 > & sig6_i', 'hls::stream< ap_uint< 128 >, 0 > & sig7_i', 'hls::stream< ap_uint< 128 >, 0 > & sig0_o', 'hls::stream< ap_uint< 128 >, 0 > & sig1_o', 'hls::stream< ap_uint< 128 >, 0 > & sig2_o', 'hls::stream< ap_uint< 128 >, 0 > & sig3_o', 'hls::stream< ap_uint< 128 >, 0 > & sig4_o', 'hls::stream< ap_uint< 128 >, 0 > & sig5_o', 'hls::stream< ap_uint< 128 >, 0 > & sig6_o', 'hls::stream< ap_uint< 128 >, 0 > & sig7_o'}  SimLibPath=''  FunctionTabVisible=on  FunctionDescription=void m16_ssr8_permute_fb_o_wrapper(hls::stream< ap_uint< 128 >, 0 > & sig0_i, hls::stream< ap_uint< 128 >, 0 > & sig1_i, hls::stream< ap_uint< 128 >, 0 > & sig2_i, hls::stream< ap_uint< 128 >, 0 > & sig3_i, hls::stream< ap_uint< 128 >, 0 > & sig4_i, hls::stream< ap_uint< 128 >, 0 > & sig5_i, hls::stream< ap_uint< 128 >, 0 > & sig6_i, hls::stream< ap_uint< 128 >, 0 > & sig7_i, hls::stream< ap_uint< 128 >, 0 > & sig0_o, hls::stream< ap_uint< 128 >, 0 > & sig1_o, hls::stream< ap_uint< 128 >, 0 > & sig2_o, hls::stream< ap_uint< 128 >, 0 > & sig3_o, hls::stream< ap_uint< 128 >, 0 > & sig4_o, hls::stream< ap_uint< 128 >, 0 > & sig5_o, hls::stream< ap_uint< 128 >, 0 > & sig6_o, hls::stream< ap_uint< 128 >, 0 > & sig7_o)  blockJsonConstraints=[]  deprecateConstraints=0  KernelHeaderFile=/proj/xcoswmktg/robg/git/designs/channelizer/hls/m16_ssr8_permute_fb_o/m16_ssr8_permute_fb_o.h  KernelFunction=m16_ssr8_permute_fb_o_wrapper  KernelFunctionSelect=<empty>  KernelSourceFile=/proj/xcoswmktg/robg/git/designs/channelizer/hls/m16_ssr8_permute_fb_o/m16_ssr8_permute_fb_o.cpp  KernelSearchPaths={}  PreProcOptions={}
  wires:
  Gain51/1 -> AIE to HLS5/1
  Signal From Workspace26/1 -> Gain49/1
  AIE to HLS6/1 -> m16_ssr8_permute_fb_i_wrapper/6
  Gain32/1 -> AIE to HLS1/1
  Gain50/1 -> AIE to HLS4/1
  Gain49/1 -> AIE to HLS3/1
  Signal From Workspace27/1 -> Gain50/1
  AIE to HLS7/1 -> m16_ssr8_permute_fb_i_wrapper/7
  Gain52/1 -> AIE to HLS6/1
  Gain53/1 -> AIE to HLS7/1
  Signal From Workspace30/1 -> Gain53/1
  m16_ssr8_permute_fb_i_wrapper/3 -> HLS to AIE10/1
  AIE to HLS2/1 -> m16_ssr8_permute_fb_i_wrapper/2
  Signal From Workspace28/1 -> Gain51/1
  m16_ssr8_permute_fb_i_wrapper/5 -> HLS to AIE12/1
  m16_ssr8_permute_fb_i_wrapper/1 -> HLS to AIE8/1
  Signal From Workspace25/1 -> Gain48/1
  AIE to HLS5/1 -> m16_ssr8_permute_fb_i_wrapper/5
  Gain48/1 -> AIE to HLS2/1
  AIE to HLS3/1 -> m16_ssr8_permute_fb_i_wrapper/3
  m16_ssr8_permute_fb_i_wrapper/7 -> HLS to AIE14/1
  Signal From Workspace29/1 -> Gain52/1
  m16_ssr8_permute_fb_i_wrapper/2 -> HLS to AIE9/1
  Signal From Workspace24/1 -> Gain32/1
  AIE to HLS1/1 -> m16_ssr8_permute_fb_i_wrapper/1
  m16_ssr8_permute_fb_i_wrapper/4 -> HLS to AIE11/1
  m16_ssr8_permute_fb_i_wrapper/8 -> HLS to AIE15/1
  AIE to HLS4/1 -> m16_ssr8_permute_fb_i_wrapper/4
  m16_ssr8_permute_fb_i_wrapper/6 -> HLS to AIE13/1
  Gain44/1 -> Variable Size Signal to Workspace18/1
  Gain45/1 -> Variable Size Signal to Workspace19/1
  Gain47/1 -> Variable Size Signal to Workspace23/1
  Gain40/1 -> Variable Size Signal to Workspace16/1
  Gain43/1 -> Variable Size Signal to Workspace21/1
  Gain41/1 -> Variable Size Signal to Workspace17/1
  Gain42/1 -> Variable Size Signal to Workspace20/1
  Gain46/1 -> Variable Size Signal to Workspace22/1
  HLS to AIE8/1 -> Gain46/1
  HLS to AIE9/1 -> Gain47/1
  HLS to AIE10/1 -> Gain40/1
  HLS to AIE11/1 -> Gain41/1
  HLS to AIE12/1 -> Gain44/1
  HLS to AIE13/1 -> Gain45/1
  HLS to AIE14/1 -> Gain42/1
  HLS to AIE15/1 -> Gain43/1
  HLS to AIE6/1 -> Gain5/1
  HLS to AIE5/1 -> Gain4/1
  HLS to AIE4/1 -> Gain7/1
  HLS to AIE3/1 -> Gain6/1
  HLS to AIE2/1 -> Gain3/1
  HLS to AIE1/1 -> Gain2/1
  HLS to AIE16/1 -> Gain9/1
  HLS to AIE7/1 -> Gain8/1
  m16_ssr8_permute_fb_o_wrapper/6 -> HLS to AIE4/1
  m16_ssr8_permute_fb_o_wrapper/8 -> HLS to AIE6/1
  m16_ssr8_permute_fb_o_wrapper/4 -> HLS to AIE2/1
  AIE to HLS8/1 -> m16_ssr8_permute_fb_o_wrapper/1
  m16_ssr8_permute_fb_o_wrapper/2 -> HLS to AIE16/1
  m16_ssr8_permute_fb_o_wrapper/7 -> HLS to AIE5/1
  Gain10/1 -> AIE to HLS9/1
  m16_ssr8_permute_fb_o_wrapper/1 -> HLS to AIE7/1
  m16_ssr8_permute_fb_o_wrapper/5 -> HLS to AIE3/1
  m16_ssr8_permute_fb_o_wrapper/3 -> HLS to AIE1/1
  Gain15/1 -> AIE to HLS14/1
  Gain14/1 -> AIE to HLS13/1
  Gain11/1 -> AIE to HLS10/1
  Gain12/1 -> AIE to HLS11/1
  Gain1/1 -> AIE to HLS8/1
  Gain13/1 -> AIE to HLS12/1
  AIE to HLS9/1 -> m16_ssr8_permute_fb_o_wrapper/2
  AIE to HLS10/1 -> m16_ssr8_permute_fb_o_wrapper/3
  AIE to HLS11/1 -> m16_ssr8_permute_fb_o_wrapper/4
  AIE to HLS12/1 -> m16_ssr8_permute_fb_o_wrapper/5
  AIE to HLS13/1 -> m16_ssr8_permute_fb_o_wrapper/6
  AIE to HLS14/1 -> m16_ssr8_permute_fb_o_wrapper/7
  AIE to HLS22/1 -> m16_ssr8_permute_fb_o_wrapper/8
  Gain31/1 -> AIE to HLS22/1
  Gain25/1 -> AIE to HLS20/1
  Signal From Workspace9/1 -> Gain25/1
  AIE to HLS20/1 -> m16_ssr8_cyclic_shift_wrapper1/8
  AIE to HLS19/1 -> m16_ssr8_cyclic_shift_wrapper1/7
  AIE to HLS18/1 -> m16_ssr8_cyclic_shift_wrapper1/6
  AIE to HLS17/1 -> m16_ssr8_cyclic_shift_wrapper1/5
  AIE to HLS16/1 -> m16_ssr8_cyclic_shift_wrapper1/4
  AIE to HLS15/1 -> m16_ssr8_cyclic_shift_wrapper1/3
  AIE to HLS23/1 -> m16_ssr8_cyclic_shift_wrapper1/2
  Gain20/1 -> AIE to HLS17/1
  Signal From Workspace11/1 -> Gain18/1
  Gain16/1 -> AIE to HLS21/1
  Gain19/1 -> AIE to HLS16/1
  Gain18/1 -> AIE to HLS15/1
  Signal From Workspace12/1 -> Gain19/1
  Gain21/1 -> AIE to HLS18/1
  Gain22/1 -> AIE to HLS19/1
  Signal From Workspace16/1 -> Gain22/1
  m16_ssr8_cyclic_shift_wrapper1/3 -> HLS to AIE17/1
  Signal From Workspace13/1 -> Gain20/1
  m16_ssr8_cyclic_shift_wrapper1/5 -> HLS to AIE20/1
  m16_ssr8_cyclic_shift_wrapper1/1 -> HLS to AIE24/1
  Signal From Workspace10/1 -> Gain17/1
  Gain17/1 -> AIE to HLS23/1
  m16_ssr8_cyclic_shift_wrapper1/7 -> HLS to AIE22/1
  Signal From Workspace14/1 -> Gain21/1
  m16_ssr8_cyclic_shift_wrapper1/2 -> HLS to AIE18/1
  Signal From Workspace8/1 -> Gain16/1
  AIE to HLS21/1 -> m16_ssr8_cyclic_shift_wrapper1/1
  m16_ssr8_cyclic_shift_wrapper1/4 -> HLS to AIE19/1
  m16_ssr8_cyclic_shift_wrapper1/8 -> HLS to AIE23/1
  m16_ssr8_cyclic_shift_wrapper1/6 -> HLS to AIE21/1
  Gain28/1 -> Variable Size Signal to Workspace11/1
  Gain29/1 -> Variable Size Signal to Workspace12/1
  Gain33/1 -> Variable Size Signal to Workspace24/1
  Gain23/1 -> Variable Size Signal to Workspace9/1
  Gain27/1 -> Variable Size Signal to Workspace14/1
  Gain24/1 -> Variable Size Signal to Workspace10/1
  Gain26/1 -> Variable Size Signal to Workspace13/1
  Gain30/1 -> Variable Size Signal to Workspace15/1
  HLS to AIE24/1 -> Gain30/1
  HLS to AIE18/1 -> Gain33/1
  HLS to AIE17/1 -> Gain23/1
  HLS to AIE19/1 -> Gain24/1
  HLS to AIE20/1 -> Gain28/1
  HLS to AIE21/1 -> Gain29/1
  HLS to AIE22/1 -> Gain26/1
  HLS to AIE23/1 -> Gain27/1
  Gain8/1 -> Variable Size Signal to Workspace7/1
  Gain9/1 -> Variable Size Signal to Workspace8/1
  Gain2/1 -> Variable Size Signal to Workspace1/1
  Gain3/1 -> Variable Size Signal to Workspace2/1
  Gain6/1 -> Variable Size Signal to Workspace3/1
  Gain7/1 -> Variable Size Signal to Workspace4/1
  Gain4/1 -> Variable Size Signal to Workspace5/1
  Gain5/1 -> Variable Size Signal to Workspace6/1
  Signal From Workspace17/1 -> Gain1/1
  Signal From Workspace18/1 -> Gain10/1
  Signal From Workspace19/1 -> Gain11/1
  Signal From Workspace20/1 -> Gain12/1
  Signal From Workspace21/1 -> Gain13/1
  Signal From Workspace22/1 -> Gain14/1
  Signal From Workspace23/1 -> Gain15/1
  Signal From Workspace31/1 -> Gain31/1
